simulink model "initialModel"  (R2023a)
settings: Solver=ode5  StartTime=0.0  StopTime=121  RelTol=1e-3
libraries: instrumentseriallib x2
settings Model: PacingRate=10  Creator=lion  LastModifiedBy=lion
settings HardwareCC: ProdBitPerLong=64  ProdHWDeviceType=Intel->x86-64 (Linux 64)
settings RTWCC: Description=Simulink Desktop Real-Time  SystemTargetFile=sldrt.tlc  TemplateMakefile=sldrt.tmf  RTWCompilerOptimization=on
settings CodeAppCC: MaxIdLength=95
settings SimulinkDesktopRealTimeCC: TargetLibSuffix=_sldrt.a  TargetPreCompLibLocation=C:\Program Files\MATLAB\R2023a\toolbox\sldrt\lib\win64

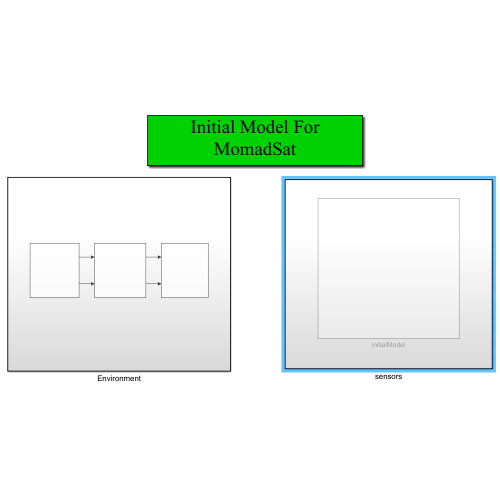
[thumbnail: Simulink's stored preview of the top-level diagram]
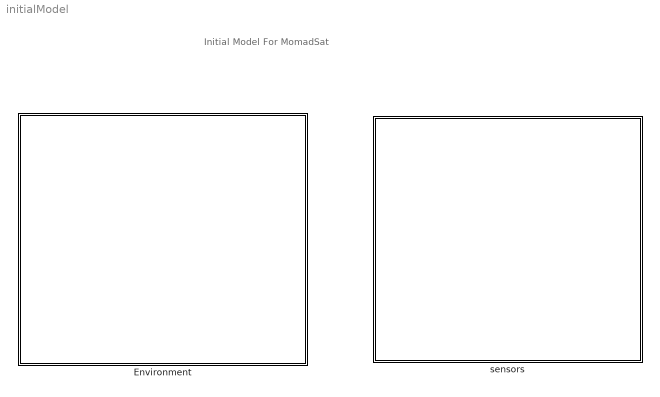
== system initialModel ==
  note: Initial Model For MomadSat
  Environment : Subsystem
  sensors : Subsystem

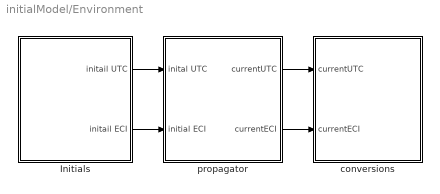
== system initialModel/Environment ==
  Initials : Subsystem
  conversions : Subsystem
  propagator : Subsystem
  wires:
  Initials/1(initail UTC) -> propagator/1(inital UTC)
  Initials/2(initail ECI) -> propagator/2(initial ECI)
  propagator/1(currentUTC) -> conversions/1(currentUTC)
  propagator/2(currentECI) -> conversions/2(currentECI)

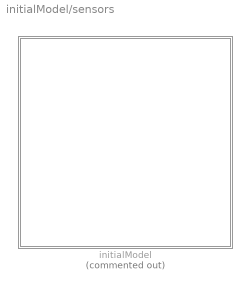
== system initialModel/sensors ==
  initialModel : Subsystem  Commented=on

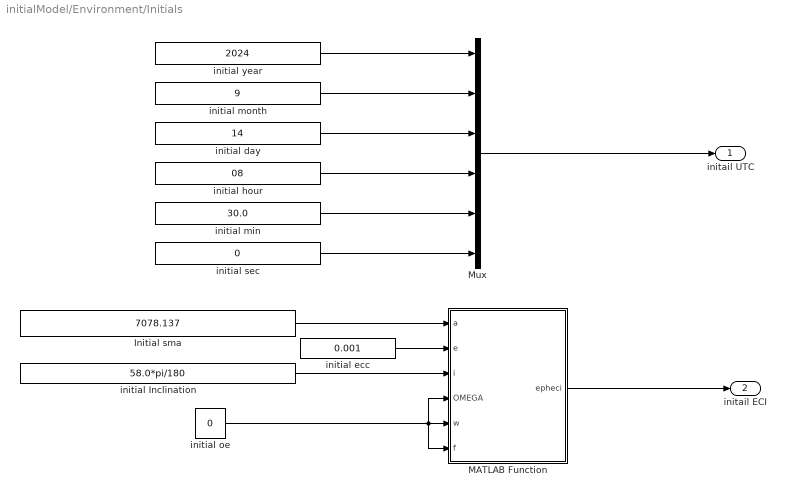
== system initialModel/Environment/Initials ==
  Initial sma : Constant  Value=7078.137
  MATLAB Function : MATLAB Function  TreatAsAtomicUnit=on
  Mux : Mux  Inputs=6
  initial Inclination : Constant  Value=58.0*pi/180
  initial day : Constant  Value=14
  initial ecc : Constant  Value=0.001
  initial hour : Constant  Value=08
  initial min : Constant  Value=30.0
  initial month : Constant  Value=9
  initial oe : Constant  Value=0
  initial sec : Constant  Value=0
  initial year : Constant  Value=2024
  initail UTC : Outport
  initail ECI : Outport  Port=2
  wires:
  initial oe/1 -> MATLAB Function/6(f), MATLAB Function/4(OMEGA), MATLAB Function/5(w)
  initial ecc/1 -> MATLAB Function/2(e)
  Initial sma/1 -> MATLAB Function/1(a)
  initial Inclination/1 -> MATLAB Function/3(i)
  initial year/1 -> Mux/1
  initial month/1 -> Mux/2
  initial day/1 -> Mux/3
  initial hour/1 -> Mux/4
  initial min/1 -> Mux/5
  initial sec/1 -> Mux/6
  Mux/1 -> initail UTC/1
  MATLAB Function/1(epheci) -> initail ECI/1

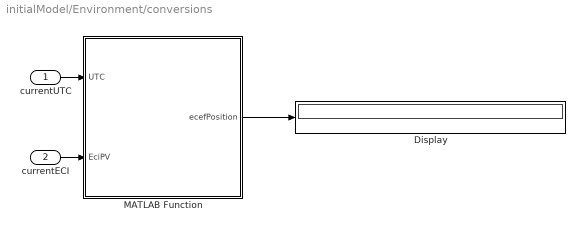
== system initialModel/Environment/conversions ==
  currentUTC : Inport
  currentECI : Inport  Port=2
  Display : Display
  MATLAB Function : MATLAB Function  TreatAsAtomicUnit=on
  wires:
  currentUTC/1 -> MATLAB Function/1(UTC)
  currentECI/1 -> MATLAB Function/2(EciPV)
  MATLAB Function/1(ecefPosition) -> Display/1

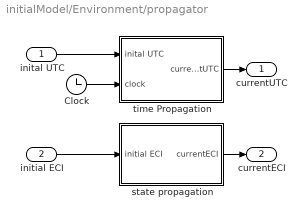
== system initialModel/Environment/propagator ==
  inital UTC : Inport
  initial ECI : Inport  Port=2
  Clock : Clock
  state propagation : Subsystem
  time Propagation : Subsystem
  currentUTC : Outport
  currentECI : Outport  Port=2
  wires:
  inital UTC/1 -> time Propagation/1(inital UTC)
  initial ECI/1 -> state propagation/1(initial ECI)
  Clock/1 -> time Propagation/2(clock)
  time Propagation/1(currentUTC) -> currentUTC/1
  state propagation/1(currentECI) -> currentECI/1

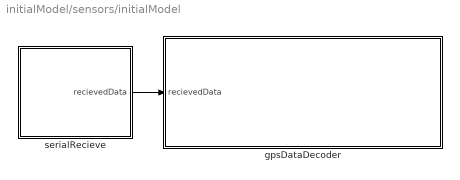
== system initialModel/sensors/initialModel ==
  gpsDataDecoder : Subsystem
  serialRecieve : Subsystem
  wires:
  serialRecieve/1(recievedData) -> gpsDataDecoder/1(recievedData)

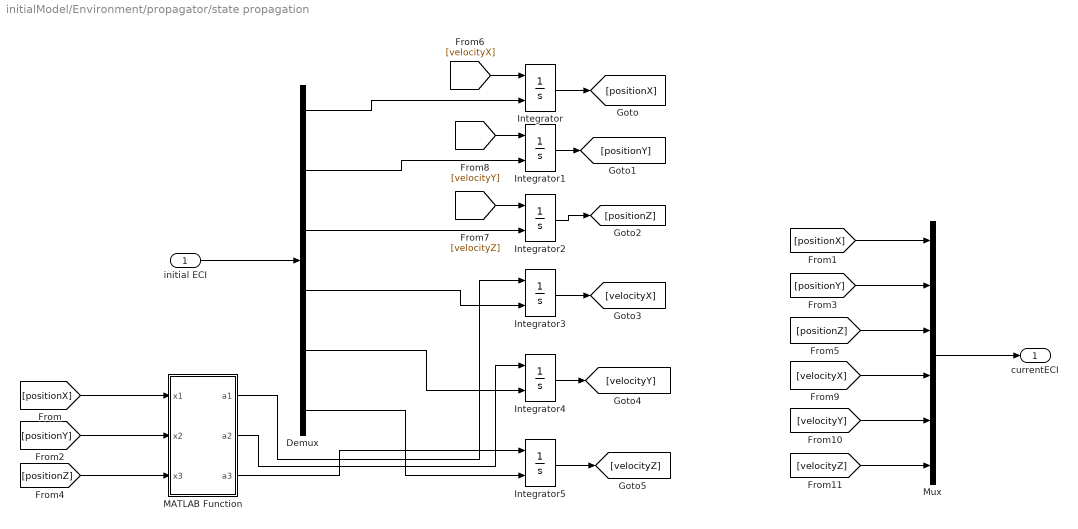
== system initialModel/Environment/propagator/state propagation ==
  initial ECI : Inport
  Demux : Demux  Outputs=6
  Integrator{,1..5} (6 alike) : Integrator  InitialConditionSource=external
  MATLAB Function : MATLAB Function  TreatAsAtomicUnit=on
  Mux : Mux  Inputs=6
  currentECI : Outport
  wires:
  Integrator3/1 -> [velocityX]
  Mux/1 -> currentECI/1
  [positionY] -> Mux/2
  Integrator/1 -> [positionX]
  Demux/6 -> Integrator5/2
  [velocityZ] -> Integrator2/1
  [positionZ] -> Mux/3
  Demux/4 -> Integrator3/2
  MATLAB Function/1(a1) -> Integrator3/1
  Integrator4/1 -> [velocityY]
  [positionX] -> MATLAB Function/1(x1)
  Demux/2 -> Integrator1/2
  Demux/3 -> Integrator2/2
  MATLAB Function/2(a2) -> Integrator4/1
  Demux/5 -> Integrator4/2
  MATLAB Function/3(a3) -> Integrator5/1
  [positionX] -> Mux/1
  Integrator1/1 -> [positionY]
  [positionY] -> MATLAB Function/2(x2)
  [positionZ] -> MATLAB Function/3(x3)
  Integrator5/1 -> [velocityZ]
  Integrator2/1 -> [positionZ]
  Demux/1 -> Integrator/2
  [velocityX] -> Integrator/1
  [velocityY] -> Integrator1/1
  initial ECI/1 -> Demux/1
  [velocityX] -> Mux/4
  [velocityY] -> Mux/5
  [velocityZ] -> Mux/6

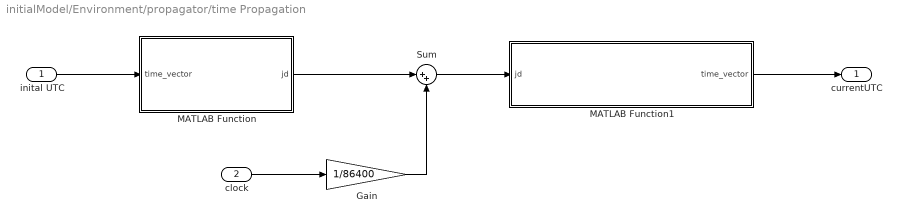
== system initialModel/Environment/propagator/time Propagation ==
  inital UTC : Inport
  clock : Inport  Port=2
  Gain : Gain  Gain=1/86400
  MATLAB Function : MATLAB Function  TreatAsAtomicUnit=on
  MATLAB Function1 : MATLAB Function  TreatAsAtomicUnit=on
  Sum : Sum  Inputs=|++
  currentUTC : Outport
  wires:
  inital UTC/1 -> MATLAB Function/1(time_vector)
  MATLAB Function1/1(time_vector) -> currentUTC/1
  MATLAB Function/1(jd) -> Sum/1
  Sum/1 -> MATLAB Function1/1(jd)
  Gain/1 -> Sum/2
  clock/1 -> Gain/1

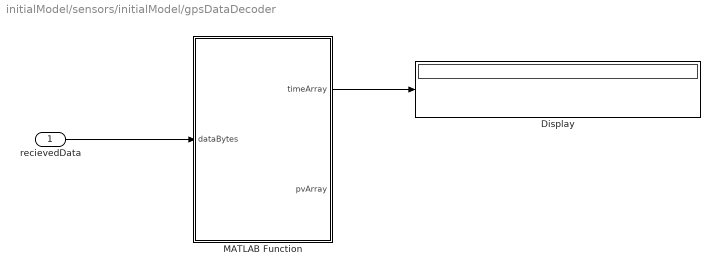
== system initialModel/sensors/initialModel/gpsDataDecoder ==
  recievedData : Inport
  Display : Display
  MATLAB Function : MATLAB Function  TreatAsAtomicUnit=on
  wires:
  recievedData/1 -> MATLAB Function/1(dataBytes)
  MATLAB Function/1(timeArray) -> Display/1

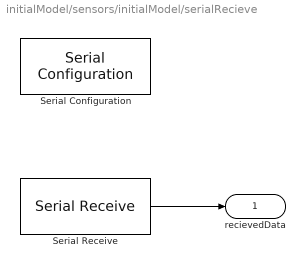
== system initialModel/sensors/initialModel/serialRecieve ==
  Serial Configuration : instrumentseriallib/Serial Configuration  Priority=-200000  PortSel=COM2  Port=COM2  ComPort=COM2  BaudRate=115200  DataBits=8  Parity=none  StopBits=1  ByteOrder=little-endian  FlowControl=none  Timeout=0.01  SimulateUsing=Interpreted execution  BlockInModel=on  aMode=1
  Serial Receive : instrumentseriallib/Serial Receive  Priority=1  PortSel=COM2  Port=COM2  ComPort=COM2  DataType=uint8  SaveDataType=uint8  ToggleHeader=on  Header=[12,21,12,21]  ToggleTerminator=on  Terminator=Custom terminator  CustomTerminator=[0,0,0,0]  InputFormat=Column major  ToggleDataSize=on  DataSize=[1 48]  EnableBlockingMode=on  ActionDataUnavailable=Output last received value  ActionWhenDataUnavailable=Output last received value  CustomValue=0  SampleTime=0.01  SimulateUsing=Interpreted execution  BlockInModel=on  aMode=1
  recievedData : Outport
  wires:
  Serial Receive/1 -> recievedData/1

== matlab function initialModel/Environment/propagator/time Propagation/MATLAB Function ==
  data: time_vector input; jd output
function jd = converToJday(time_vector)
jd = 367.0 * time_vector(1)  ...
    - floor( (7 * (time_vector(1) + floor( (time_vector(2) + 9) / 12.0) ) ) * 0.25 )   ...
    + floor( 275 * time_vector(2) / 9.0 ) ...
    + time_vector(3) + 1721013.5;
jdfrac = (time_vector(6) + time_vector(5) * 60.0 + time_vector(4) *3600.0) / 86400.0;
% check jdfrac
if jdfrac > 1.0
    jd = jd + floor(jdfrac);
    jdfrac = jdfrac - floor(jdfrac);
end
jd = jd + jdfrac;
end

== matlab function initialModel/Environment/Initials/MATLAB Function ==
  data: a input; epheci output; e input; i input; OMEGA input; w input; f input
function epheci = convertToEci(a, e, i, OMEGA, w, f)
Trans = zeros(3, 3);
mu  = 398600.4415;
epheci = zeros(1, 6);
X = zeros(3, 1);
V = zeros(3, 1);
% a = initialCoe(1, 1);
% e = initialCoe(1, 2);
% i = initialCoe(1, 3) * pi / 180;
% OMEGA = initialCoe(1, 4) * pi / 180;
% w = initialCoe(1, 5) * pi / 180;
% f = initialCoe(1, 6) * pi / 180;
% Handle special cases:
% Circular equitorial orbit.
if e == 0 && i == 0
    w = 0;
    OMEGA = 0;
    % Circular inclined orbit.
elseif e == 0
    w = 0;
    % Elliptical equitorial.
elseif i == 0
    OMEGA = 0;
end
% Compute the semi-latus rectum.
p = a*(1-e^2);
% % Convert mean anomaly to true anomaly.
% % First, compute the eccentric anomaly.
% Ea = Keplers_Eqn(M, e);
%
% % Compute the true anomaly f.
% y = sin(Ea)*sqrt(1-e^2)/(1-e*cos(Ea));
% x = (cos(Ea)-e)/(1-e*cos(Ea));
%
% f = atan2(y,x);
% Define the position vector in perifocal PQW coordinates.
X(1,1) = p*cos(f)/(1+e*cos(f));
X(2,1) = p*sin(f)/(1+e*cos(f));
X(3,1) = 0;
% Define the velocity vector in perifocal PQW coordinates.
V(1,1) = -sqrt(mu/p)*sin(f);
V(2,1) =  sqrt(mu/p)*(e+cos(f));
V(3,1) =  0;
% Define Transformation Matrix To IJK.
Trans(1,1) =  cos(OMEGA)*cos(w)-sin(OMEGA)*sin(w)*cos(i);
Trans(1,2) = -cos(OMEGA)*sin(w)-sin(OMEGA)*cos(w)*cos(i);
Trans(1,3) =  sin(OMEGA)*sin(i);
Trans(2,1) =  sin(OMEGA)*cos(w)+cos(OMEGA)*sin(w)*cos(i);
Trans(2,2) = -sin(OMEGA)*sin(w)+cos(OMEGA)*cos(w)*cos(i);
Trans(2,3) = -cos(OMEGA)*sin(i);
Trans(3,1) =  sin(w)*sin(i);
Trans(3,2) =  cos(w)*sin(i);
Trans(3,3) =  cos(i);
% Transform to the ECI coordinate system.
X = Trans*X;
V = Trans*V;
epheci(1, 1:6) = [X',V'];
end

== matlab function initialModel/Environment/propagator/time Propagation/MATLAB Function1 ==
  data: jd input; time_vector output
function time_vector = convertToUtc(jd)
z = fix(jd + 0.5);
fday = jd + 0.5 - z;
if (fday < 0)
   fday = fday + 1;
   z = z - 1;
end
if (z < 2299161)
   a = z;
else
   alpha = floor((z - 1867216.25) / 36524.25);
   a = z + 1 + alpha - floor(alpha / 4);
end
b = a + 1524;
c = fix((b - 122.1) / 365.25);
d = fix(365.25 * c);
e = fix((b - d) / 30.6001);
day = b - d - fix(30.6001 * e) + fday;
if (e < 14)
   month = e - 1;
else
   month = e - 13;
end
if (month > 2)
   year = c - 4716;
else
   year = c - 4715;
end
hr = abs(day-floor(day))*24;
min = abs(hr-floor(hr))*60;
if min-floor(min) > 0.9999
    min = round(min);
end
sec = abs(min-floor(min))*60;
day = floor(day);
hr = floor(hr);
min = floor(min);
time_vector = [year, month, day, hr, min, sec];
end

== matlab function initialModel/Environment/propagator/state propagation/MATLAB Function ==
  data: x1 input; a1 output; x2 input; x3 input; a2 output; a3 output
function [a1,a2,a3] = gravityJ2(x1,x2,x3)
Re  = 6378.137;
J2  = 1.08262668e-3;
mu  = 398600.4415;
r   = norm([x1, x2, x3]);
a1 = -mu*x1/r^3*(1+1.5*J2*(Re/r)^2*(1-5*(x3/r)^2));
a2 = -mu*x2/r^3*(1+1.5*J2*(Re/r)^2*(1-5*(x3/r)^2));
a3 = -mu*x3/r^3*(1+1.5*J2*(Re/r)^2*(3-5*(x3/r)^2));
end

== matlab function initialModel/Environment/conversions/MATLAB Function ==
  data: UTC input; ecefPosition output; EciPV input
function ecefPosition = convertToECEF(UTC, EciPV)
%Gets the Direction Cosine Matrix for conversion between ECI and ECEF
%   Input: UTC time (6x1)
%   Output: DCM matrix (3x3)
year =  UTC(1);
mes =   UTC(2);
dia   = UTC(3);
hora  = UTC(4);
minuto= UTC(5);
segundo=UTC(6);
%1: get modified julian day (mjd)
mjd = 367*year + dia - 712269 + fix(275*mes/9)- fix(7*(year+fix((mes+9)/12))/4);
%2: get fraction of the day (dfra)
dfra = segundo + 60*(minuto + 60*hora);
%3: get Greenwich Sidereal Time (GWST)
tsj = (mjd-18262.5)/36525;
tsgo = (24110.54841 + (8640184.812866 + 9.3104e-2*tsj - 6.2e-6*tsj*tsj)*tsj)*pi/43200;
tetp = 7.292116e-5;		% Earth angular velocity (rad/s)
gwst = mod(tsgo + dfra*tetp, 2*pi);
%4: get DCM from ECI to ECEF
coan    =  cos(gwst);
sian    =  sin(gwst);
DCM_eci2ecef =  [coan, sian, 0; -sian, coan, 0; 0, 0, 1];
eciPos = EciPV(1:3)';
ecefPosition = eciPos * DCM_eci2ecef;
end

== matlab function initialModel/sensors/initialModel/gpsDataDecoder/MATLAB Function ==
  data: dataBytes input; timeArray output; pvArray output
function [timeArray, pvArray] = fcn(dataBytes)
timeArray = single(zeros(1,6));
pvArray = single(zeros(1,6));
year = typecast(dataBytes(1:4),'single');
month = typecast(dataBytes(5:8),'single');
day = typecast(dataBytes(9:12),'single');
hour = typecast(dataBytes(13:16),'single');
minute = typecast(dataBytes(17:20),'single');
second = typecast(dataBytes(21:24),'single');
posX = typecast(dataBytes(25:28),'single');
posY = typecast(dataBytes(29:32),'single');
posZ = typecast(dataBytes(33:36),'single');
velX = typecast(dataBytes(37:40),'single');
velY = typecast(dataBytes(41:44),'single');
velZ = typecast(dataBytes(45:48),'single');
pvArray = [posX, posY, posZ, velX, velY, velZ];
timeArray = [year, month, day, hour, minute, second];
end
